simulink model "sysgenFloatingPointIIR_DFormII"  (Simulink 7.5)
settings: Solver=VariableStepDiscrete  SolverMode=SingleTasking  StartTime=0.0  StopTime=500  RelTol=1e-3
PreLoadFcn:
  | xlrequire('PreLoadFcn');
InitFcn:
  | xlIIRFilterResponse;
values from neighbouring files (symbols this model uses):
  Fs = 1 ./ block_data.params.XIncr    [sdspfscope2_r13.m]
undefined symbols (not defined in the file or in its folder): DEN2, DEN3, NUM1, NUM3, One, sided, sysgen_scale, xlIIRFilterResponse
libraries: xbsIndex_r4 x23, xbsCopyrightNotice_r4 x1, dspsnks4 x1
settings Model: Creator=harinar  LastModifiedBy=arvinds

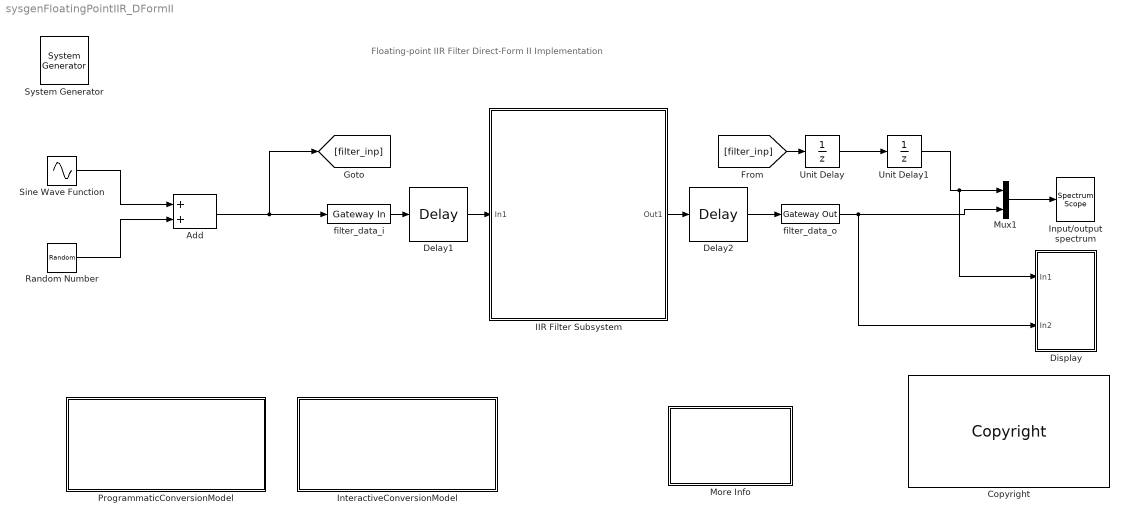
== system sysgenFloatingPointIIR_DFormII ==
  note: Floating-point IIR Filter Direct-Form II Implementation
  " System Generator" : xbsIndex_r4/ System Generator  Tag=genX  SystemSampleTime=-1  xilinxfamily=virtex6  part=xc6vsx475t  speed=-2  package=ff1156  synthesis_tool=XST  clock_wrapper=Clock Enables  directory=./netlist  proj_type=Project Navigator  Synth_file=XST Defaults  Impl_file=ISE Defaults  testbench=off  simulink_period=1/(sysgen_scale*Fs)  sysclk_period=10  dcm_input_clock_period=10  incr_netlist=off  trim_vbits=Everywhere in SubSystem  dbl_ovrd=According to Block Masks  core_generation=According to Block Masks  run_coregen=off  deprecated_control=off  eval_field=0  block_type=sysgen
      settings: block_version=13.3
  Add : Sum
  Copyright : xbsCopyrightNotice_r4/Copyright  copyrighttext="Copyright (c) 2011  by  Xilinx, Inc. All rights reserved.<br><br>This file contains proprietary, confidential information of Xilinx, Inc., is distributed under license from Xilinx, Inc., and may be used, copied and/or disclosed only pursuant to the terms of a valid license agreement with Xilinx, Inc. Xilinx hereby grants you a license to use this file solely for design, simulation, implementation and creation of design files limited to Xilinx devices or technologies. Use with non-Xilinx devices or technologies is expressly prohibited and immediately terminates your license unless covered by a separate agreement.<br><br>Xilinx is providing this design, code, or information \"as-is\" solely for use in developing programs and solutions for Xilinx devices, with no obligation on the part of Xilinx to provide support. By providing this design, code, or information as one possible implementation of this feature, application or standard, Xilinx is making no representation that this implementation is free from any claims of infringement. You are responsible for obtaining any rights you may require for your implementation. Xilinx expressly disclaims any warranty whatsoever with respect to the adequacy of the implementation, including but not limited to any warranties or representations that this implementation is free from claims of infringement, implied warranties of merchantability or fitness for a particular purpose.<br><br>Xilinx products are not intended for use in life support appliances, devices, or systems. Use in such applications is expressly prohibited.<br><br>Any modifications that are made to the Source Code are done at the user's sole risk and will be unsupported.<br><br>This copyright and support notice must be retained as part of this text at all times. (c) Copyright 1995-2011 Xilinx, Inc. All rights reserved."  block_type=copyright
      settings: block_version=10.1.00
  Delay1 : xbsIndex_r4/Delay  rst=off  infoeditControl=Selection of Reset will increase slice count due to use of real FFs and instead of SRLs  en=off  latency=1  dbl_ovrd=off  reg_retiming=off  block_type=delay
      settings: block_version=13.3
  Delay2 : xbsIndex_r4/Delay  rst=off  infoeditControl=Selection of Reset will increase slice count due to use of real FFs and instead of SRLs  en=off  latency=1  dbl_ovrd=off  reg_retiming=off  block_type=delay
      settings: block_version=13.3
  Display : Subsystem
  IIR Filter Subsystem : Subsystem
  Input/output spectrum : dspsnks4/Spectrum Scope  DialogController=dspdialog.SpectrumScope  DialogControllerArgs=DataTag1  SystemSampleTime=-1  ScopeProperties=off  Domain=Frequency  HorizSpan=1  UseBuffer=on  BufferSize=512  Overlap=0  inpFftLenInherit=off  FFTlength=128  numAvg=1  DisplayProperties=off  AxisGrid=on  Memory=off  FrameNumber=on  AxisLegend=off  AxisZoom=off  OpenScopeAtSimStart=on  OpenScopeImmediately=off  FigPos=[1105 390 423 236]  AxisProperties=off  XUnits=Hertz  XRange=One-sided ([0...Fs/2])  XDisplay=0  InheritXIncr=off  XIncr=1/Fs  XLabel=Samples  XLimit=Auto  YUnits=dBW/Hertz  XMax=1  XMin=0  YLabel=Magnitude, dB  LineProperties=off  LineColors=[0.1 0.2 0.7]|[0.6 0.2 0.1]|[0.1 0.6 0.1]  wintypeSpecScope=Hann  RsSpecScope=50  betaSpecScope=5  winsampSpecScope=Periodic  XAxisParamsVer=6.9
      settings: YMin=-100  YMax=0
  InteractiveConversionModel : Subsystem
      settings: OpenFcn=xlConvertModel_I();
      mask Display: disp('Double click\n  to\n  switch between\n  Fixed-point and Floating-point\n  interactively');
  More Info : Subsystem
      mask Display: disp('Double click\n for\n more information.')
  Mux1 : Mux  Inputs=2
  ProgrammaticConversionModel : Subsystem
      settings: OpenFcn=xlConvertModel_P();
      mask Display: disp('Double click\n  to\n  switch between\n  Fixed-point and Floating-point\n  programmatically');
  Random Number : RandomNumber  Variance=10  SampleTime=1/(Fs)
  Sine Wave Function : Sin  Amplitude=1  Bias=0  Frequency=2*3.14*5000  Phase=0  Samples=10  SampleTime=1/(Fs)  Offset=0
  Unit Delay : UnitDelay  SampleTime=-1
  Unit Delay1 : UnitDelay  SampleTime=-1
  filter_data_i : xbsIndex_r4/Gateway In  gui_display_data_type=Floating-point  arith_type=Floating-point  n_bits=32  bin_pt=24  preci_type=Custom  exp_width=6  frac_width=9  quantization="Round  (unbiased: +/- Inf)"  overflow=Saturate  period=1/(Fs)  dbl_ovrd=off  timing_constraint=None  locs_specified=off  LOCs={}  hdl_port=on  block_type=gatewayin
      settings: infoedit="Gateway in block.  Converts inputs of type Simulink integer, double and fixed point to  Xilinx fixed point or floating-point data type.<br><br>Hardware notes:  In hardware these blocks become top level input ports."  block_version=13.3
  filter_data_o : xbsIndex_r4/Gateway Out  hdl_port=on  timing_constraint=None  locs_specified=off  LOCs={}  block_type=gatewayout
      settings: infoedit="Gateway out block.  Converts Xilinx fixed point inputs into ouputs of type Simulink integer, double, or fixed point.<br><br>Hardware notes:  In hardware these blocks become top level output ports or are discarded, depending on how they are configured."  block_version=13.3
  wires:
  IIR Filter Subsystem/1(Out1) -> Delay2/1
  Sine Wave Function/1 -> Add/1
  filter_data_i/1 -> Delay1/1
  Random Number/1 -> Add/2
  Add/1 -> filter_data_i/1, [filter_inp]
  Mux1/1 -> Input/output spectrum/1
  [filter_inp] -> Unit Delay/1
  filter_data_o/1 -> Mux1/2, Display/2(In2)
  Delay1/1 -> IIR Filter Subsystem/1(In1)
  Delay2/1 -> filter_data_o/1
  Unit Delay/1 -> Unit Delay1/1
  Unit Delay1/1 -> Mux1/1, Display/1(In1)

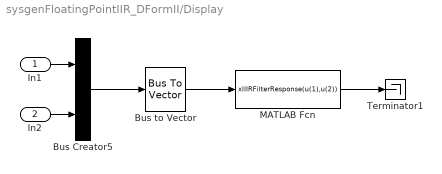
== system sysgenFloatingPointIIR_DFormII/Display ==
  In1 : Inport
  In2 : Inport  Port=2
  Bus Creator5 : BusCreator  Inputs=2
  Bus to Vector : BusToVector
  MATLAB Fcn : MATLABFcn  MATLABFcn=xlIIRFilterResponse(u(1),u(2))
  Terminator1 : Terminator
  wires:
  MATLAB Fcn/1 -> Terminator1/1
  Bus to Vector/1 -> MATLAB Fcn/1
  Bus Creator5/1 -> Bus to Vector/1
  In1/1 -> Bus Creator5/1
  In2/1 -> Bus Creator5/2

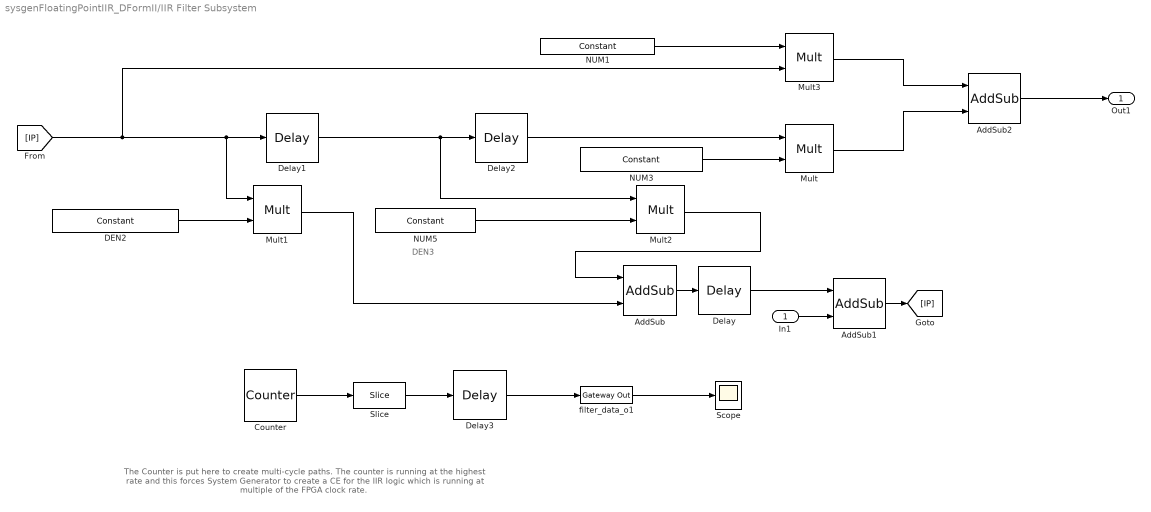
== system sysgenFloatingPointIIR_DFormII/IIR Filter Subsystem ==
  note: DEN3
  note: The Counter is put here to create multi-cycle paths. The counter is running at the highest rate
      | and this forces System Generator  to create a CE for the IIR logic which is running at multiple of  the
      | FPGA clock rate.
  In1 : Inport
  AddSub : xbsIndex_r4/AddSub  mode=Addition  use_carryin=off  use_carryout=off  en=off  latency=0  precision=Full  arith_type="Signed  (2's comp)"  n_bits=32  bin_pt=24  quantization=Truncate  overflow=Wrap  dbl_ovrd=off  use_behavioral_HDL=off  hw_selection=DSP48  pipelined=off  block_type=addsub
      settings: block_version=13.3
  AddSub1 : xbsIndex_r4/AddSub  mode=Addition  use_carryin=off  use_carryout=off  en=off  latency=0  precision=Full  arith_type="Signed  (2's comp)"  n_bits=32  bin_pt=24  quantization=Truncate  overflow=Wrap  dbl_ovrd=off  use_behavioral_HDL=off  hw_selection=DSP48  pipelined=off  block_type=addsub
      settings: block_version=13.3
  AddSub2 : xbsIndex_r4/AddSub  mode=Addition  use_carryin=off  use_carryout=off  en=off  latency=0  precision=Full  arith_type="Signed  (2's comp)"  n_bits=32  bin_pt=24  quantization=Truncate  overflow=Wrap  dbl_ovrd=off  use_behavioral_HDL=off  hw_selection=DSP48  pipelined=off  block_type=addsub
      settings: block_version=13.3
  Counter : xbsIndex_r4/Counter  cnt_type=Free Running  cnt_to=Inf  operation=Up  start_count=0  cnt_by_val=1  arith_type=Unsigned  n_bits=4  bin_pt=0  load_pin=off  rst=off  en=off  explicit_period=on  period=1/(sysgen_scale*Fs)  dbl_ovrd=off  use_behavioral_HDL=off  implementation=Fabric  block_type=counter
      settings: block_version=13.3
  DEN2 : xbsIndex_r4/Constant  const=DEN2  gui_display_data_type=Floating-point  arith_type=Floating-point  n_bits=32  bin_pt=24  preci_type=Custom  exp_width=6  frac_width=9  explicit_period=on  period=1/(Fs)  equ=P=C  opselect=C  inp2=PCIN>>17  opr=+  inp1=P  carry=CIN  dbl_ovrd=off  block_type=constant
      settings: block_version=13.3
  Delay{,1..3} (4 alike) : xbsIndex_r4/Delay  rst=off  infoeditControl=Selection of Reset will increase slice count due to use of real FFs and instead of SRLs  en=off  latency=1  dbl_ovrd=off  reg_retiming=off  block_type=delay
      settings: block_version=13.3
  Mult{,1..3} (4 alike) : xbsIndex_r4/Mult  precision=Full  arith_type="Signed  (2's comp)"  n_bits=32  bin_pt=24  quantization=Truncate  overflow=Wrap  en=off  latency=0  dbl_ovrd=off  use_behavioral_HDL=off  opt=Speed  use_embedded=on  optimum_pipeline=off  pipeline=on  use_rpm=on  placement_style=Triangular  block_type=mult
      settings: block_version=13.3
  NUM1 : xbsIndex_r4/Constant  const=NUM1  gui_display_data_type=Floating-point  arith_type=Floating-point  n_bits=32  bin_pt=24  preci_type=Custom  exp_width=6  frac_width=9  explicit_period=on  period=1/(Fs)  equ=P=C  opselect=C  inp2=PCIN>>17  opr=+  inp1=P  carry=CIN  dbl_ovrd=off  block_type=constant
      settings: block_version=13.3
  NUM3 : xbsIndex_r4/Constant  const=NUM3  gui_display_data_type=Floating-point  arith_type=Floating-point  n_bits=32  bin_pt=24  preci_type=Custom  exp_width=6  frac_width=9  explicit_period=on  period=1/(Fs)  equ=P=C  opselect=C  inp2=PCIN>>17  opr=+  inp1=P  carry=CIN  dbl_ovrd=off  block_type=constant
      settings: block_version=13.3
  NUM5 : xbsIndex_r4/Constant  const=DEN3  gui_display_data_type=Floating-point  arith_type=Floating-point  n_bits=32  bin_pt=24  preci_type=Custom  exp_width=6  frac_width=9  explicit_period=on  period=1/(Fs)  equ=P=C  opselect=C  inp2=PCIN>>17  opr=+  inp1=P  carry=CIN  dbl_ovrd=off  block_type=constant
      settings: block_version=13.3
  Scope : Scope
  Slice : xbsIndex_r4/Slice  nbits=4  boolean_output=off  mode=Upper Bit Location + Width  bit1=0  base1=MSB of Input  bit0=0  base0=LSB of Input  dbl_ovrd=off  block_type=slice
      settings: block_version=13.3
  filter_data_o1 : xbsIndex_r4/Gateway Out  hdl_port=off  timing_constraint=None  locs_specified=off  LOCs={}  block_type=gatewayout
      settings: infoedit="Gateway out block.  Converts Xilinx fixed point or floating-point type inputs into ouputs of type Simulink integer, double, or fixed point.<br><br>Hardware notes:  In hardware these blocks become top level output ports or are discarded, depending on how they are configured."  block_version=13.3
  Out1 : Outport
  wires:
  Delay1/1 -> Mult2/1, Delay2/1
  NUM3/1 -> Mult/2
  DEN2/1 -> Mult1/2
  NUM5/1 -> Mult2/2
  Mult1/1 -> AddSub/2
  Mult2/1 -> AddSub/1
  NUM1/1 -> Mult3/1
  Mult3/1 -> AddSub2/1
  Mult/1 -> AddSub2/2
  [IP] -> Mult3/2, Delay1/1, Mult1/1
  AddSub2/1 -> Out1/1
  AddSub1/1 -> [IP]
  AddSub/1 -> Delay/1
  In1/1 -> AddSub1/2
  Delay/1 -> AddSub1/1
  Delay2/1 -> Mult/1
  Counter/1 -> Slice/1
  filter_data_o1/1 -> Scope/1
  Slice/1 -> Delay3/1
  Delay3/1 -> filter_data_o1/1

== system sysgenFloatingPointIIR_DFormII/InteractiveConversionModel ==

== system sysgenFloatingPointIIR_DFormII/More Info ==
  note: Floating-point IIR Filter Direct-Form II Implementation
  note: This design is a model for Direct Form II realization of a second-order IIR Filter (Peaking Filter).
      |
      | The design shows Sysgen's capability to switch between Floating point and Fixed point data.
      |
      | The same design can be modified to a Fixed-point model -
      |         a) Programmatically, using the 'ConversionModel' switch present at the top-level or
      |         b) Manually, by configuring different blocks in the system (a brief description available at the top-level)
      |
      | It can be noticed from the plotted filter-reponses, using a Floating-point system (Custom precision, Exponent-width=6, Fraction-width=9) it
      | achieves a  much better filter-response with less-than-half the total-bitwidth, when compared to the Fixed-point model (Number of bits = 32,
      | Binary point = 24).
      |
      | Implementation notes:
      |
      | For Floating-point system:
      | - Input precision ('Arithmetic type', 'Number of bits' and 'Binary point') at the GatewayIn and Constant block-GUIs should be same.
      | - Output precision at the Addsub and Multiplier blocks should be selected as 'Full' precision.
      |
      | For Fixed-point system:
      | -  Output precision ('Output type', 'Number of bits' and 'Binary point') at the Addsub and Multiplier block-GUIs should be specified explicitly,
      |     by selecting 'User defined' precision.
      |
      | The operating clock frequency for the top-level design as shown is 48KHz and input signal-frequency is 5KHz and SNR being ~ -13dB.
      |
      | At the top-level system, a counter is added to create multi-cycle paths. The counter is running at the highest rate and this forces
      | System Generator to create a CE for the IIR logic which is running at a multiple of  the FPGA clock rate.

== system sysgenFloatingPointIIR_DFormII/ProgrammaticConversionModel ==
